simulink model "plant_harness"  (R2021a)
settings: Solver=ode4  StartTime=0.0  StopTime=10.0  FixedStep=0.001  RelTol=1e-3
undefined symbols (not defined in the file): DiscIntNeverNeededParam
libraries: vrlib x8, dspinverses x2, simulink x1, aerolibutil x1
settings Model: NumberOfSteps=10  Creator=jadg1  LastModifiedBy=jadg1

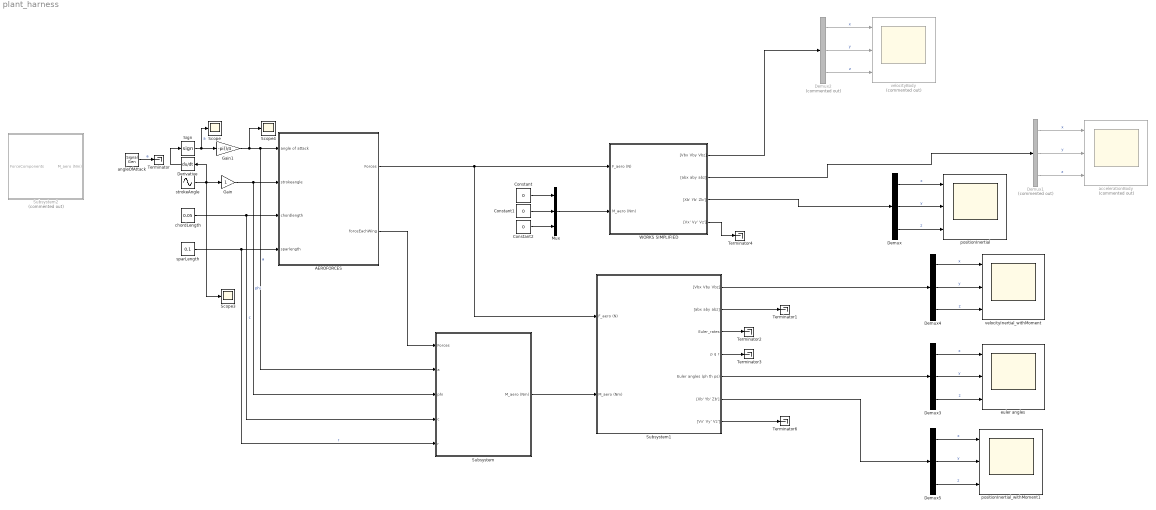
== system plant_harness ==
  AEROFORCES : Subsystem
  Constant : Constant  Value=0
  Constant1 : Constant  Value=0
  Constant2 : Constant  Value=0
  Demux{,3..5} (4 alike) : Demux  Outputs=3
  Demux1 : Demux  Commented=on  Outputs=3
  Demux2 : Demux  Commented=on  Outputs=3
  Derivative : Derivative
  Gain : Gain
  Gain1 : Gain  Gain=-pi()/4
  Mux : Mux  Inputs=3
  Scope : Scope
  Scope3 : Scope
  Scope4 : Scope
  Sign : Signum
  Subsystem : Subsystem
  Subsystem1 : Subsystem
  Subsystem2 : Subsystem  Commented=on
  Terminator{,1..4,6} (6 alike) : Terminator
  WORKS SIMPLIFIED : Subsystem
  accelerationBody : Scope  Commented=on  NumInputPorts=3
  angleOfAttack : SignalGenerator  WaveForm=square  Amplitude=pi()/6  Frequency=30
  chordLength : Constant  Value=0.05
  euler angles : Scope  NumInputPorts=3
  positionInertial : Scope  NumInputPorts=3
  positionInertial_withMoment1 : Scope  NumInputPorts=3
  sparLength : Constant  Value=0.1
  strokeAngle : Sin  Amplitude=pi()/2  Frequency=20*2*pi  Phase=pi()/2  SampleTime=0
  velocityBody : Scope  Commented=on  NumInputPorts=3
  velocityInertial_withMoment : Scope  NumInputPorts=3
  wires:
  sparLength/1 -> Subsystem/5(r), AEROFORCES/4(sparlength)  "r"
  chordLength/1 -> Subsystem/4(c), AEROFORCES/3(chordlength)  "c"
  Mux/1 -> WORKS SIMPLIFIED/2(M_aero (Nm))
  WORKS SIMPLIFIED/3("[Xb' Yb' Zb']") -> Demux/1
  WORKS SIMPLIFIED/4("[Vx' Vy' Vz']") -> Terminator4/1
  strokeAngle/1 -> Derivative/1, Scope3/1, Gain/1
  WORKS SIMPLIFIED/2("[abx aby abz]") -> Demux1/1
  WORKS SIMPLIFIED/1("[Vbx Vby Vbz]") -> Demux2/1
  Sign/1 -> Scope/1, Gain1/1  "a"
  Constant1/1 -> Mux/2
  Constant/1 -> Mux/1
  Constant2/1 -> Mux/3
  Demux/1 -> positionInertial/1  "x"
  Demux/2 -> positionInertial/2  "y"
  Demux/3 -> positionInertial/3  "z"
  Demux1/3 -> accelerationBody/3  "z"
  Demux1/2 -> accelerationBody/2  "y"
  Demux1/1 -> accelerationBody/1  "x"
  Demux2/1 -> velocityBody/1  "x"
  Demux2/2 -> velocityBody/2  "y"
  Demux2/3 -> velocityBody/3  "z"
  Demux3/3 -> euler angles/3  "z"
  Demux3/2 -> euler angles/2  "y"
  Demux3/1 -> euler angles/1  "x"
  Subsystem1/5(Euler angles (ph th ps)) -> Demux3/1
  Subsystem1/1("[Vbx Vby Vbz]") -> Demux4/1
  Subsystem1/2("[abx aby abz]") -> Terminator1/1
  Subsystem1/7("[Vx' Vy' Vz']") -> Terminator6/1
  Demux4/1 -> velocityInertial_withMoment/1  "x"
  Demux4/2 -> velocityInertial_withMoment/2  "y"
  Demux4/3 -> velocityInertial_withMoment/3  "z"
  Gain/1 -> Subsystem/3(phi), AEROFORCES/2(strokeangle)  "phi"
  Demux5/1 -> positionInertial_withMoment1/1  "x"
  Demux5/2 -> positionInertial_withMoment1/2  "y"
  Demux5/3 -> positionInertial_withMoment1/3  "z"
  Subsystem1/6("[Xb' Yb' Zb']") -> Demux5/1
  Subsystem1/3(Euler_rates) -> Terminator2/1
  Subsystem1/4(p q r) -> Terminator3/1
  Subsystem/1(M_aero (Nm)) -> Subsystem1/2(M_aero (Nm))
  AEROFORCES/2(forceEachWing) -> Subsystem/1(Forces)
  Gain1/1 -> Scope4/1, Subsystem/2(a), AEROFORCES/1(angle of attack)  "a"
  angleOfAttack/1 -> Terminator/1  "a"
  Derivative/1 -> Sign/1
  AEROFORCES/1(Forces) -> Subsystem1/1(F_aero (N)), WORKS SIMPLIFIED/1(F_aero (N))

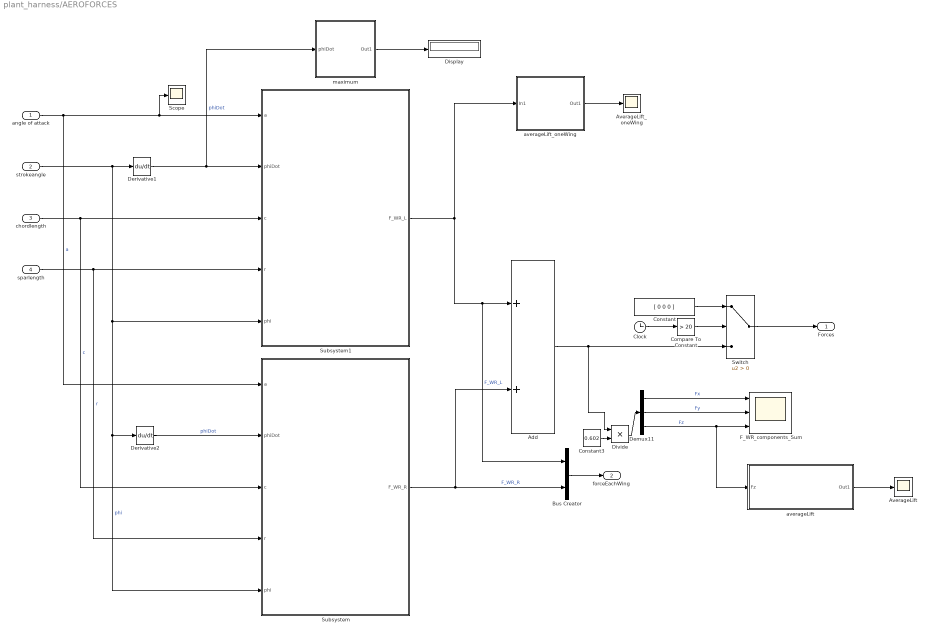
== system plant_harness/AEROFORCES ==
  angle of attack : Inport
  strokeangle : Inport  Port=2
  chordlength : Inport  Port=3
  sparlength : Inport  Port=4
  Add : Sum
  AverageLift : Scope
  AverageLift_oneWing : Scope
  Bus Creator : BusCreator  Inputs=2
  Clock : Clock
  Compare To Constant : simulink/Logic and Bit Operations/Compare To Constant  relop=>  const=20  OutDataTypeStr=boolean
  Constant : Constant  Value=[ 0 0 0 ]
  Constant3 : Constant  Value=0.602
  Demux11 : Demux  Outputs=3
  Derivative1 : Derivative
  Derivative2 : Derivative
  Display : Display
  Divide : Product  Inputs=**
  F_WR_components_Sum : Scope  NumInputPorts=3
  Scope : Scope
  Subsystem : Subsystem
  Subsystem1 : Subsystem
  Switch : Switch  Criteria=u2 > Threshold
  averageLift : Subsystem
  averageLift_oneWing : Subsystem
  maximum : Subsystem
  Forces : Outport
  forceEachWing : Outport  Port=2
  wires:
  Derivative1/1 -> maximum/1(phiDot), Subsystem1/2(phiDot)  "phiDot"
  Add/1 -> Divide/1, Switch/3
  Demux11/1 -> F_WR_components_Sum/1  "Fx"
  Demux11/3 -> F_WR_components_Sum/3, averageLift/1(Fz)  "Fz"
  Demux11/2 -> F_WR_components_Sum/2  "Fy"
  strokeangle/1 -> Subsystem/5(phi), Derivative2/1, Subsystem1/5(phi), Derivative1/1  "phi"
  chordlength/1 -> Subsystem/3(c), Subsystem1/3(c)  "c"
  sparlength/1 -> Subsystem/4(r), Subsystem1/4(r)  "r"
  Derivative2/1 -> Subsystem/2(phiDot)  "phiDot"
  Subsystem/1(F_WR_R) -> Add/2, Bus Creator/2  "F_WR_R"
  angle of attack/1 -> Subsystem/1(a), Scope/1, Subsystem1/1(a)  "a"
  Subsystem1/1(F_WR_L) -> averageLift_oneWing/1(In1), Bus Creator/1, Add/1  "F_WR_L"
  averageLift_oneWing/1(Out1) -> AverageLift_oneWing/1
  averageLift/1(Out1) -> AverageLift/1
  maximum/1(Out1) -> Display/1
  Switch/1 -> Forces/1
  Clock/1 -> Compare To Constant/1
  Compare To Constant/1 -> Switch/2
  Constant/1 -> Switch/1
  Bus Creator/1 -> forceEachWing/1
  Constant3/1 -> Divide/2
  Divide/1 -> Demux11/1

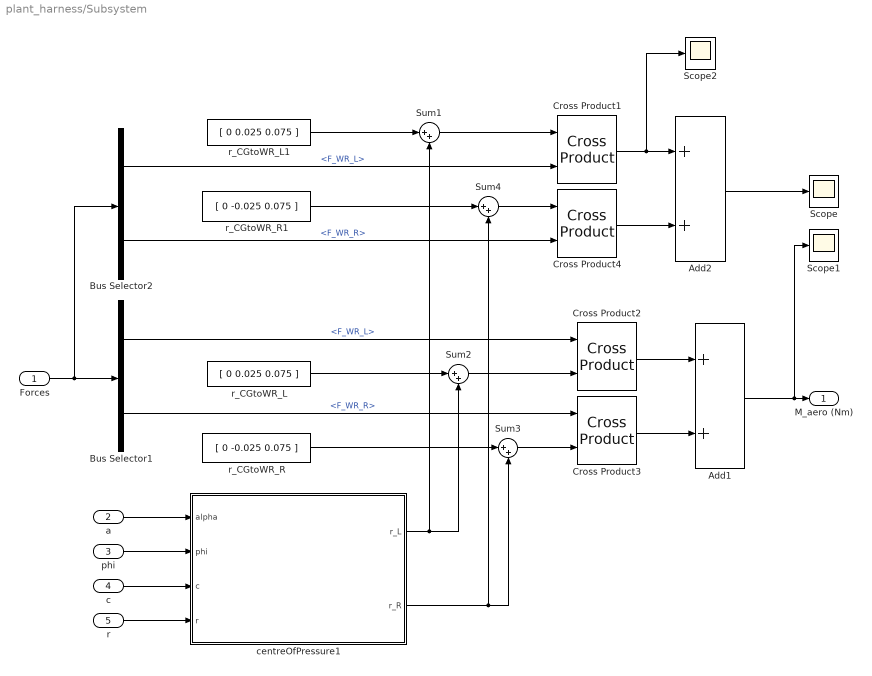
== system plant_harness/Subsystem ==
  Forces : Inport
  a : Inport  Port=2
  phi : Inport  Port=3
  c : Inport  Port=4
  r : Inport  Port=5
  Add1 : Sum
  Add2 : Sum
  Bus Selector1 : BusSelector  OutputSignals=F_WR_L,F_WR_R
  Bus Selector2 : BusSelector  OutputSignals=F_WR_L,F_WR_R
  Cross Product{1..4} (4 alike) : vrlib/Utilities/Cross Product
  Scope : Scope
  Scope1 : Scope
  Scope2 : Scope
  Sum{1..4} (4 alike) : Sum  Inputs=|++
  centreOfPressure1 : MATLAB Function  TreatAsAtomicUnit=on
  r_CGtoWR_L : Constant  Value=[ 0 0.025 0.075 ]
  r_CGtoWR_L1 : Constant  Value=[ 0 0.025 0.075 ]
  r_CGtoWR_R : Constant  Value=[ 0 -0.025 0.075 ]
  r_CGtoWR_R1 : Constant  Value=[ 0 -0.025 0.075 ]
  M_aero (Nm) : Outport
  wires:
  Bus Selector1/1 -> Cross Product2/1  "<F_WR_L>"
  r_CGtoWR_R/1 -> Sum3/1
  phi/1 -> centreOfPressure1/2(phi)
  centreOfPressure1/2(r_R) -> Sum4/2, Sum3/2
  Sum2/1 -> Cross Product2/2
  centreOfPressure1/1(r_L) -> Sum1/2, Sum2/2
  r/1 -> centreOfPressure1/4(r)
  c/1 -> centreOfPressure1/3(c)
  Sum3/1 -> Cross Product3/2
  Bus Selector1/2 -> Cross Product3/1  "<F_WR_R>"
  Add1/1 -> Scope1/1, M_aero (Nm)/1
  a/1 -> centreOfPressure1/1(alpha)
  Cross Product3/1 -> Add1/2
  Cross Product2/1 -> Add1/1
  Forces/1 -> Bus Selector2/1, Bus Selector1/1
  r_CGtoWR_L/1 -> Sum2/1
  Cross Product1/1 -> Scope2/1, Add2/1
  Cross Product4/1 -> Add2/2
  Bus Selector2/2 -> Cross Product4/2  "<F_WR_R>"
  Bus Selector2/1 -> Cross Product1/2  "<F_WR_L>"
  Sum1/1 -> Cross Product1/1
  r_CGtoWR_L1/1 -> Sum1/1
  Sum4/1 -> Cross Product4/1
  r_CGtoWR_R1/1 -> Sum4/1
  Add2/1 -> Scope/1

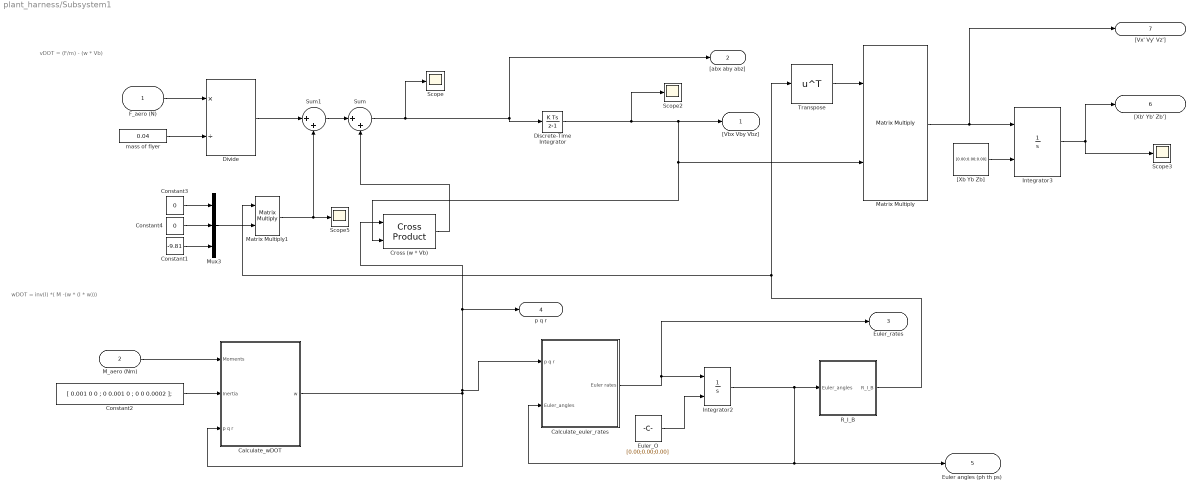
== system plant_harness/Subsystem1 ==
  note: wDOT = inv(I) *( M -(w * (I * w)))
  note: vDOT = (F/m) - (w * Vb)
  F_aero (N) : Inport
  M_aero (Nm) : Inport  Port=2
  Calculate_euler_rates : Subsystem
  Calculate_wDOT : Subsystem
  Constant1 : Constant  Value=-9.81
  Constant2 : Constant  Value=[ 0.001 0 0 ; 0 0.001 0 ; 0 0 0.0002 ];
  Constant3 : Constant  Value=0
  Constant4 : Constant  Value=0
  Cross (w * Vb) : vrlib/Utilities/Cross Product
  Discrete-Time Integrator : DiscreteIntegrator  SampleTime=-1  ICPrevOutput=DiscIntNeverNeededParam  ICPrevScaledInput=DiscIntNeverNeededParam
  Divide : Product  Inputs=*/
  Euler_O : Constant  Value=[0.00;0.00;0.00]
  Integrator2 : Integrator  InitialConditionSource=external
  Integrator3 : Integrator  InitialConditionSource=external
  Matrix Multiply : Product  Multiplication=Matrix(*)
  Matrix Multiply1 : Product  Multiplication=Matrix(*)
  Mux3 : Mux  Inputs=3
  R_I_B : Subsystem
  Scope{,2..3,5} (4 alike) : Scope
  Sum : Sum  Inputs=|++
  Sum1 : Sum  Inputs=|++
  Transpose : Math  Operator=transpose  SaturateOnIntegerOverflow=on
  "[Xb Yb Zb]" : Constant  Value=[0.00;0.00;0.00]
  mass of flyer : Constant  Value=0.04
  "[Vbx Vby Vbz]" : Outport
  "[abx aby abz]" : Outport  Port=2
  Euler_rates : Outport  Port=3
  p q r : Outport  Port=4
  Euler angles (ph th ps) : Outport  Port=5
  "[Xb' Yb' Zb']" : Outport  Port=6
  "[Vx' Vy' Vz']" : Outport  Port=7
  wires:
  Euler_O/1 -> Integrator2/2
  M_aero (Nm)/1 -> Calculate_wDOT/1(Moments)
  Calculate_euler_rates/1(Euler rates) -> Euler_rates/1, Integrator2/1
  F_aero (N)/1 -> Divide/1
  Transpose/1 -> Matrix Multiply/1
  "[Xb Yb Zb]"/1 -> Integrator3/2
  mass of flyer/1 -> Divide/2
  Calculate_wDOT/1(w) -> Calculate_wDOT/3(p q r), Cross (w * Vb)/1, p q r/1, Calculate_euler_rates/1(p q r)
  Constant2/1 -> Calculate_wDOT/2(Inertia)
  Matrix Multiply/1 -> "[Vx' Vy' Vz']"/1, Integrator3/1
  Discrete-Time Integrator/1 -> Scope2/1, "[Vbx Vby Vbz]"/1, Cross (w * Vb)/2, Matrix Multiply/2
  Integrator3/1 -> Scope3/1, "[Xb' Yb' Zb']"/1
  Cross (w * Vb)/1 -> Sum/2
  Integrator2/1 -> Calculate_euler_rates/2(Euler_angles), Euler angles (ph th ps)/1, R_I_B/1(Euler_angles)
  Sum/1 -> Scope/1, "[abx aby abz]"/1, Discrete-Time Integrator/1
  Constant4/1 -> Mux3/2
  Mux3/1 -> Matrix Multiply1/2
  Constant3/1 -> Mux3/1
  Matrix Multiply1/1 -> Sum1/2, Scope5/1
  Constant1/1 -> Mux3/3
  R_I_B/1(R_I_B) -> Matrix Multiply1/1, Transpose/1
  Divide/1 -> Sum1/1
  Sum1/1 -> Sum/1

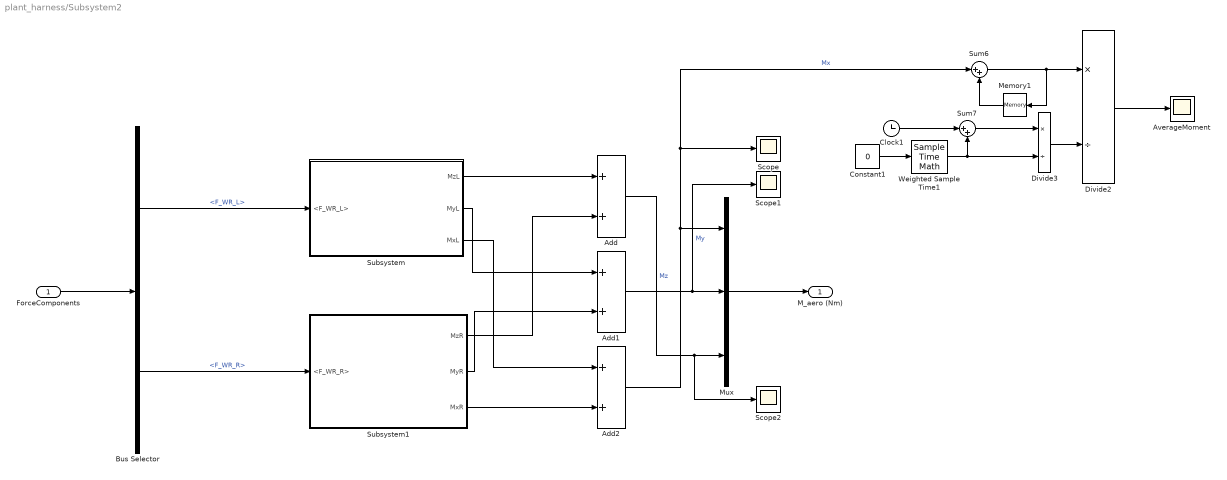
== system plant_harness/Subsystem2 ==
  ForceComponents : Inport
  Add : Sum
  Add1 : Sum
  Add2 : Sum
  AverageMoment : Scope
  Bus Selector : BusSelector  OutputSignals=F_WR_L,F_WR_R
  Clock1 : Clock
  Constant1 : Constant  Value=0
  Divide2 : Product  Inputs=*/
  Divide3 : Product  Inputs=*/
  Memory1 : Memory
  Mux : Mux  Inputs=3
  Scope : Scope
  Scope1 : Scope
  Scope2 : Scope
  Subsystem : Subsystem
  Subsystem1 : Subsystem
  Sum6 : Sum  Inputs=|++
  Sum7 : Sum  Inputs=|++
  Weighted Sample Time1 : SampleTimeMath  TsampMathOp=Ts Only
  M_aero (Nm) : Outport
  wires:
  ForceComponents/1 -> Bus Selector/1
  Bus Selector/1 -> Subsystem/1(<F_WR_L>)  "<F_WR_L>"
  Bus Selector/2 -> Subsystem1/1(<F_WR_R>)  "<F_WR_R>"
  Subsystem1/1(MzR) -> Add/2
  Subsystem/1(MzL) -> Add/1
  Subsystem1/2(MyR) -> Add1/2
  Subsystem/2(MyL) -> Add1/1
  Subsystem1/3(MxR) -> Add2/2
  Subsystem/3(MxL) -> Add2/1
  Add2/1 -> Sum6/1, Scope/1, Mux/1  "Mx"
  Add/1 -> Scope2/1, Mux/3  "Mz"
  Add1/1 -> Scope1/1, Mux/2  "My"
  Mux/1 -> M_aero (Nm)/1
  Weighted Sample Time1/1 -> Sum7/2, Divide3/2
  Sum6/1 -> Memory1/1, Divide2/1
  Constant1/1 -> Weighted Sample Time1/1
  Clock1/1 -> Sum7/1
  Divide3/1 -> Divide2/2
  Sum7/1 -> Divide3/1
  Divide2/1 -> AverageMoment/1
  Memory1/1 -> Sum6/2

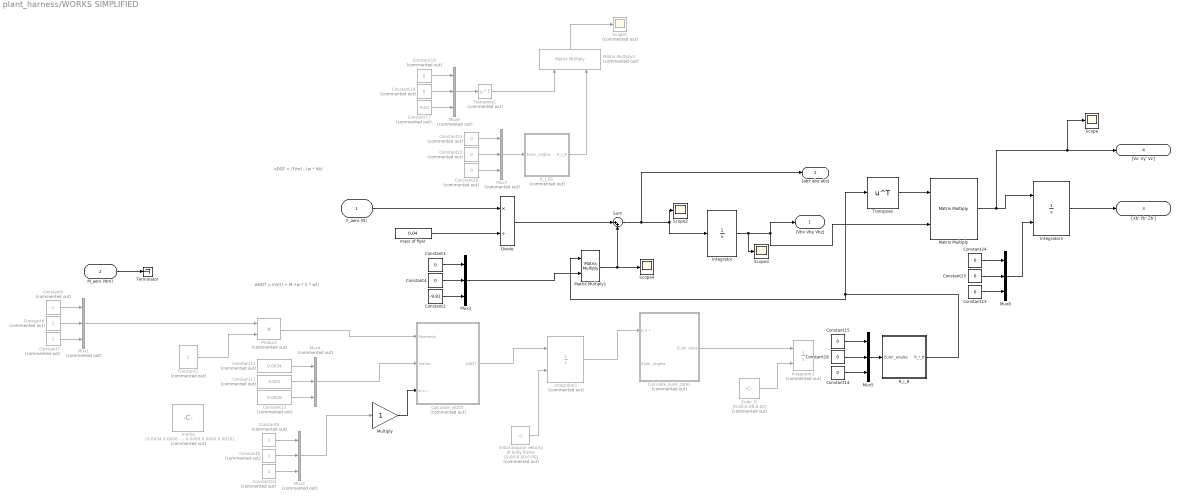
== system plant_harness/WORKS SIMPLIFIED ==
  note: wDOT = inv(I) + M -(w * (I * w))
  note: vDOT = (F/m) - (w * Vb)
  F_aero (N) : Inport
  M_aero (Nm) : Inport  Port=2
  Calculate_euler_rates : Subsystem  Commented=on
  Calculate_wDOT : Subsystem  Commented=on
  Constant{1,5..10} (7 alike) : Constant  Commented=on
  Constant11 : Constant  Commented=on  Value=0.001
  Constant12 : Constant  Commented=on  Value=0.0034
  Constant13 : Constant  Commented=on  Value=0.0026
  Constant{3..4,14..16,23..25} (8 alike) : Constant  Value=0
  Constant17 : Constant  Commented=on  Value=-9.81
  Constant{18..22} (5 alike) : Constant  Commented=on  Value=0
  Constant2 : Constant  Value=-9.81
  Divide : Product  Inputs=*/
  Euler_O : Constant  Commented=on  Value=[0.00;0.00;0.00]
  Inertia : Constant  Commented=on  Value=[0.0034 0.0000 0.0000; 0.0000 0.0010 0.0000; 0.0000 0.0000 0.0026]
  Initial angular velocity of body frame : Constant  Commented=on  Value=[0.00;0.00;0.00]
  Integrator : Integrator
  Integrator1 : Integrator  Commented=on  InitialConditionSource=external
  Integrator2 : Integrator  Commented=on  InitialConditionSource=external
  Integrator3 : Integrator  InitialConditionSource=external
  Matrix Multiply : Product  Multiplication=Matrix(*)
  Matrix Multiply1 : Product  Multiplication=Matrix(*)
  Matrix Multiply2 : Product  Commented=on  Multiplication=Matrix(*)
  Multiply : Gain
  Mux{1..2,4,6..7} (5 alike) : Mux  Commented=on  Inputs=3
  Mux3 : Mux  Inputs=3
  Mux5 : Mux  Inputs=3
  Mux8 : Mux  Inputs=3
  Product : Product  Commented=on
  R_I_B : Subsystem
  R_I_B1 : Subsystem  Commented=on
  Scope{,2..4} (4 alike) : Scope
  Scope1 : Scope  Commented=on
  Sum : Sum  Inputs=|++
  Terminator : Terminator
  Transpose : Math  Operator=transpose  SaturateOnIntegerOverflow=on
  Transpose1 : Math  Commented=on  Operator=transpose  SaturateOnIntegerOverflow=on
  mass of flyer : Constant  Value=0.04
  "[Vbx Vby Vbz]" : Outport
  "[abx aby abz]" : Outport  Port=2
  "[Xb' Yb' Zb']" : Outport  Port=3
  "[Vx' Vy' Vz']" : Outport  Port=4
  wires:
  mass of flyer/1 -> Divide/2
  M_aero (Nm)/1 -> Terminator/1
  Constant8/1 -> Mux2/1
  Euler_O/1 -> Integrator2/2
  Constant9/1 -> Mux2/2
  Product/1 -> Calculate_wDOT/1(Moments)
  F_aero (N)/1 -> Divide/1
  Constant13/1 -> Mux4/3
  Transpose/1 -> Matrix Multiply/1
  Initial angular velocity of body frame/1 -> Integrator1/2
  Integrator/1 -> Scope3/1, Matrix Multiply/2, "[Vbx Vby Vbz]"/1
  Integrator1/1 -> Calculate_euler_rates/1(p q r)
  Constant10/1 -> Mux2/3
  Mux4/1 -> Calculate_wDOT/2(Inertia)
  Constant12/1 -> Mux4/1
  Calculate_euler_rates/1(Euler rates) -> Integrator2/1
  Constant11/1 -> Mux4/2
  Mux2/1 -> Multiply/1
  Multiply/1 -> Calculate_wDOT/3(p q r)
  Matrix Multiply/1 -> "[Vx' Vy' Vz']"/1, Scope/1, Integrator3/1
  R_I_B/1(R_I_B) -> Transpose/1, Matrix Multiply1/1
  Constant1/1 -> Product/2
  Calculate_wDOT/1(wDOT) -> Integrator1/1
  Constant5/1 -> Mux1/1
  Constant6/1 -> Mux1/2
  Mux1/1 -> Product/1
  Constant7/1 -> Mux1/3
  Integrator3/1 -> "[Xb' Yb' Zb']"/1
  Constant16/1 -> Mux5/2
  Constant15/1 -> Mux5/1
  Mux5/1 -> R_I_B/1(Euler_angles)
  Constant14/1 -> Mux5/3
  Divide/1 -> Sum/1
  Sum/1 -> "[abx aby abz]"/1, Scope2/1, Integrator/1
  Constant2/1 -> Mux3/3
  Constant3/1 -> Mux3/1
  Constant4/1 -> Mux3/2
  Constant18/1 -> Mux6/1
  Constant19/1 -> Mux6/2
  Constant17/1 -> Mux6/3
  Constant20/1 -> Mux7/3
  Constant21/1 -> Mux7/1
  Constant22/1 -> Mux7/2
  Matrix Multiply2/1 -> Scope1/1
  Mux7/1 -> R_I_B1/1(Euler_angles)
  Mux6/1 -> Transpose1/1
  Transpose1/1 -> Matrix Multiply2/1
  R_I_B1/1(R_I_B) -> Matrix Multiply2/2
  Matrix Multiply1/1 -> Scope4/1, Sum/2
  Mux3/1 -> Matrix Multiply1/2
  Mux8/1 -> Integrator3/2
  Constant23/1 -> Mux8/3
  Constant25/1 -> Mux8/2
  Constant24/1 -> Mux8/1

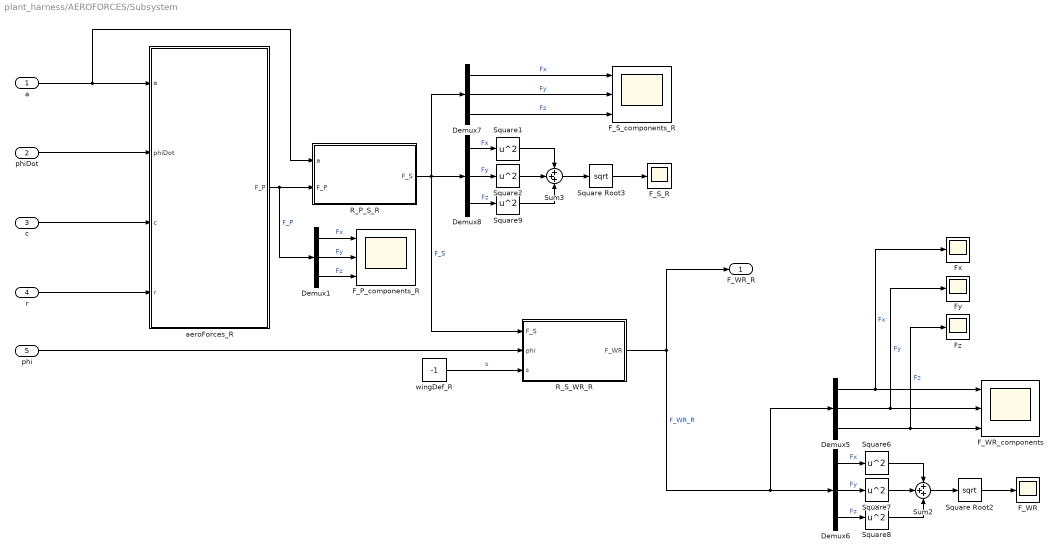
== system plant_harness/AEROFORCES/Subsystem ==
  a : Inport
  phiDot : Inport  Port=2
  c : Inport  Port=3
  r : Inport  Port=4
  phi : Inport  Port=5
  Demux{1,5..8} (5 alike) : Demux  Outputs=3
  F_P_components_R : Scope  NumInputPorts=3
  F_S_R : Scope
  F_S_components_R : Scope  NumInputPorts=3
  F_WR : Scope
  F_WR_components : Scope  NumInputPorts=3
  Fx : Scope
  Fy : Scope
  Fz : Scope
  R_P_S_R : MATLAB Function  TreatAsAtomicUnit=on
  R_S_WR_R : MATLAB Function  TreatAsAtomicUnit=on
  Square Root2 : Sqrt  SaturateOnIntegerOverflow=on
  Square Root3 : Sqrt  SaturateOnIntegerOverflow=on
  Square{1..2,6..9} (6 alike) : Math  Operator=square  SaturateOnIntegerOverflow=on
  Sum2 : Sum  Inputs=+++
  Sum3 : Sum  Inputs=+++
  aeroForces_R : MATLAB Function  TreatAsAtomicUnit=on
  wingDef_R : Constant  Value=-1
  F_WR_R : Outport
  wires:
  Demux8/3 -> Square9/1  "Fz"
  Square9/1 -> Sum3/3
  aeroForces_R/1(F_P) -> R_P_S_R/2(F_P), Demux1/1  "F_P"
  a/1 -> aeroForces_R/1(a), R_P_S_R/1(a)
  R_P_S_R/1(F_S) -> Demux8/1, Demux7/1, R_S_WR_R/1(F_S)  "F_S"
  r/1 -> aeroForces_R/4(r)
  Demux8/1 -> Square1/1  "Fx"
  phi/1 -> R_S_WR_R/2(phi)
  Square1/1 -> Sum3/1
  Demux8/2 -> Square2/1  "Fy"
  Demux7/3 -> F_S_components_R/3  "Fz"
  Demux7/2 -> F_S_components_R/2  "Fy"
  Demux1/2 -> F_P_components_R/2  "Fy"
  Demux1/1 -> F_P_components_R/1  "Fx"
  c/1 -> aeroForces_R/3(c)
  Demux7/1 -> F_S_components_R/1  "Fx"
  Sum3/1 -> Square Root3/1
  phiDot/1 -> aeroForces_R/2(phiDot)
  Square2/1 -> Sum3/2
  Demux1/3 -> F_P_components_R/3  "Fz"
  Square Root3/1 -> F_S_R/1
  wingDef_R/1 -> R_S_WR_R/3(s)  "s"
  R_S_WR_R/1(F_WR) -> Demux5/1, Demux6/1, F_WR_R/1  "F_WR_R"
  Square Root2/1 -> F_WR/1
  Demux5/3 -> Fz/1, F_WR_components/3  "Fz"
  Demux5/2 -> F_WR_components/2, Fy/1  "Fy"
  Square7/1 -> Sum2/2
  Square8/1 -> Sum2/3
  Demux5/1 -> Fx/1, F_WR_components/1  "Fx"
  Sum2/1 -> Square Root2/1
  Demux6/2 -> Square7/1  "Fy"
  Square6/1 -> Sum2/1
  Demux6/1 -> Square6/1  "Fx"
  Demux6/3 -> Square8/1  "Fz"

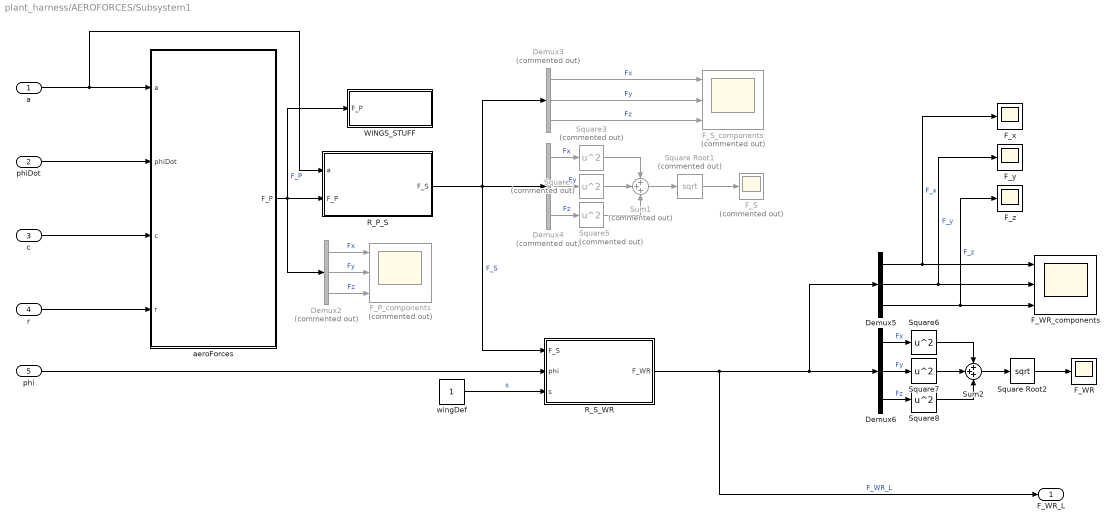
== system plant_harness/AEROFORCES/Subsystem1 ==
  a : Inport
  phiDot : Inport  Port=2
  c : Inport  Port=3
  r : Inport  Port=4
  phi : Inport  Port=5
  Demux2 : Demux  Commented=on  Outputs=3
  Demux3 : Demux  Commented=on  Outputs=3
  Demux4 : Demux  Commented=on  Outputs=3
  Demux5 : Demux  Outputs=3
  Demux6 : Demux  Outputs=3
  F_P_components : Scope  Commented=on  NumInputPorts=3
  F_S : Scope  Commented=on
  F_S_components : Scope  Commented=on  NumInputPorts=3
  F_WR : Scope
  F_WR_components : Scope  NumInputPorts=3
  F_x : Scope
  F_y : Scope
  F_z : Scope
  R_P_S : MATLAB Function  TreatAsAtomicUnit=on
  R_S_WR : MATLAB Function  TreatAsAtomicUnit=on
  Square Root1 : Sqrt  Commented=on  SaturateOnIntegerOverflow=on
  Square Root2 : Sqrt  SaturateOnIntegerOverflow=on
  Square3 : Math  Commented=on  Operator=square  SaturateOnIntegerOverflow=on
  Square4 : Math  Commented=on  Operator=square  SaturateOnIntegerOverflow=on
  Square5 : Math  Commented=on  Operator=square  SaturateOnIntegerOverflow=on
  Square6 : Math  Operator=square  SaturateOnIntegerOverflow=on
  Square7 : Math  Operator=square  SaturateOnIntegerOverflow=on
  Square8 : Math  Operator=square  SaturateOnIntegerOverflow=on
  Sum1 : Sum  Commented=on  Inputs=+++
  Sum2 : Sum  Inputs=+++
  WINGS_STUFF : Subsystem
  aeroForces : MATLAB Function  TreatAsAtomicUnit=on
  wingDef : Constant
  F_WR_L : Outport
  wires:
  Demux2/3 -> F_P_components/3  "Fz"
  wingDef/1 -> R_S_WR/3(s)  "s"
  Square6/1 -> Sum2/1
  phiDot/1 -> aeroForces/2(phiDot)
  Square7/1 -> Sum2/2
  Demux6/3 -> Square8/1  "Fz"
  Demux4/3 -> Square5/1  "Fz"
  aeroForces/1(F_P) -> WINGS_STUFF/1(F_P), Demux2/1, R_P_S/2(F_P)  "F_P"
  Demux2/1 -> F_P_components/1  "Fx"
  Demux5/3 -> F_z/1, F_WR_components/3  "F_z"
  Demux6/1 -> Square6/1  "Fx"
  Demux3/3 -> F_S_components/3  "Fz"
  R_S_WR/1(F_WR) -> F_WR_L/1, Demux5/1, Demux6/1  "F_WR_L"
  R_P_S/1(F_S) -> R_S_WR/1(F_S), Demux3/1, Demux4/1  "F_S"
  Demux3/2 -> F_S_components/2  "Fy"
  Square4/1 -> Sum1/2
  Demux6/2 -> Square7/1  "Fy"
  r/1 -> aeroForces/4(r)
  Sum2/1 -> Square Root2/1
  Demux5/1 -> F_x/1, F_WR_components/1  "F_x"
  Demux4/2 -> Square4/1  "Fy"
  Square8/1 -> Sum2/3
  Square5/1 -> Sum1/3
  Demux5/2 -> F_WR_components/2, F_y/1  "F_y"
  Square3/1 -> Sum1/1
  a/1 -> R_P_S/1(a), aeroForces/1(a)
  Square Root1/1 -> F_S/1
  Demux3/1 -> F_S_components/1  "Fx"
  Demux2/2 -> F_P_components/2  "Fy"
  Sum1/1 -> Square Root1/1
  Demux4/1 -> Square3/1  "Fx"
  Square Root2/1 -> F_WR/1
  c/1 -> aeroForces/3(c)
  phi/1 -> R_S_WR/2(phi)

== system plant_harness/AEROFORCES/averageLift ==
  Fz : Inport
  Clock : Clock
  Constant : Constant  Value=0
  Divide : Product  Inputs=*/
  Divide1 : Product  Inputs=*/
  Memory : Memory
  Sum : Sum  Inputs=|++
  Sum5 : Sum  Inputs=|++
  Weighted Sample Time : SampleTimeMath  TsampMathOp=Ts Only
  Out1 : Outport
  wires:
  Sum/1 -> Memory/1, Divide/1
  Weighted Sample Time/1 -> Sum5/2, Divide1/2
  Memory/1 -> Sum/2
  Divide1/1 -> Divide/2
  Fz/1 -> Sum/1
  Divide/1 -> Out1/1
  Constant/1 -> Weighted Sample Time/1
  Clock/1 -> Sum5/1
  Sum5/1 -> Divide1/1

== system plant_harness/AEROFORCES/averageLift_oneWing ==
  In1 : Inport
  Clock1 : Clock
  Constant1 : Constant  Value=0
  Divide2 : Product  Inputs=*/
  Divide3 : Product  Inputs=*/
  Memory1 : Memory
  Sum6 : Sum  Inputs=|++
  Sum7 : Sum  Inputs=|++
  Weighted Sample Time1 : SampleTimeMath  TsampMathOp=Ts Only
  Out1 : Outport
  wires:
  Weighted Sample Time1/1 -> Sum7/2, Divide3/2
  Sum7/1 -> Divide3/1
  Clock1/1 -> Sum7/1
  Divide3/1 -> Divide2/2
  Constant1/1 -> Weighted Sample Time1/1
  Sum6/1 -> Memory1/1, Divide2/1
  Memory1/1 -> Sum6/2
  Divide2/1 -> Out1/1
  In1/1 -> Sum6/1

== system plant_harness/AEROFORCES/maximum ==
  phiDot : Inport
  GreaterThan : RelationalOperator  Operator=>  OutDataTypeStr=boolean  RndMeth=Simplest
  Memory2 : Memory
  Switch : Switch  Criteria=u2 > Threshold
  Out1 : Outport
  wires:
  Switch/1 -> Out1/1, Memory2/1
  phiDot/1 -> GreaterThan/1, Switch/1
  Memory2/1 -> Switch/3, GreaterThan/2
  GreaterThan/1 -> Switch/2

== system plant_harness/Subsystem1/Calculate_euler_rates ==
  note: psi dot
  note: theta dot
  note: phi dot
  note: psi
  p q r : Inport
  Euler_angles : Inport  Port=2
  Calc_my_euler_rates : MATLAB Function  TreatAsAtomicUnit=on
  Demux : Demux  Outputs=[-1;1;1]
  Demux1 : Demux  Outputs=[1;1;1]
  Demux2 : Demux  Outputs=3
  Mux : Mux  Inputs=3
  Terminator : Terminator
  Euler rates : Outport
  wires:
  Demux/1 -> Terminator/1
  Euler_angles/1 -> Demux/1
  Demux/2 -> Calc_my_euler_rates/1(theta)
  Demux/3 -> Calc_my_euler_rates/2(phi)
  p q r/1 -> Demux1/1
  Demux1/2 -> Calc_my_euler_rates/4(q)
  Demux1/1 -> Calc_my_euler_rates/3(p)
  Demux1/3 -> Calc_my_euler_rates/5(r)
  Calc_my_euler_rates/1(euler_rates) -> Demux2/1
  Demux2/2 -> Mux/2
  Demux2/1 -> Mux/1
  Demux2/3 -> Mux/3
  Mux/1 -> Euler rates/1

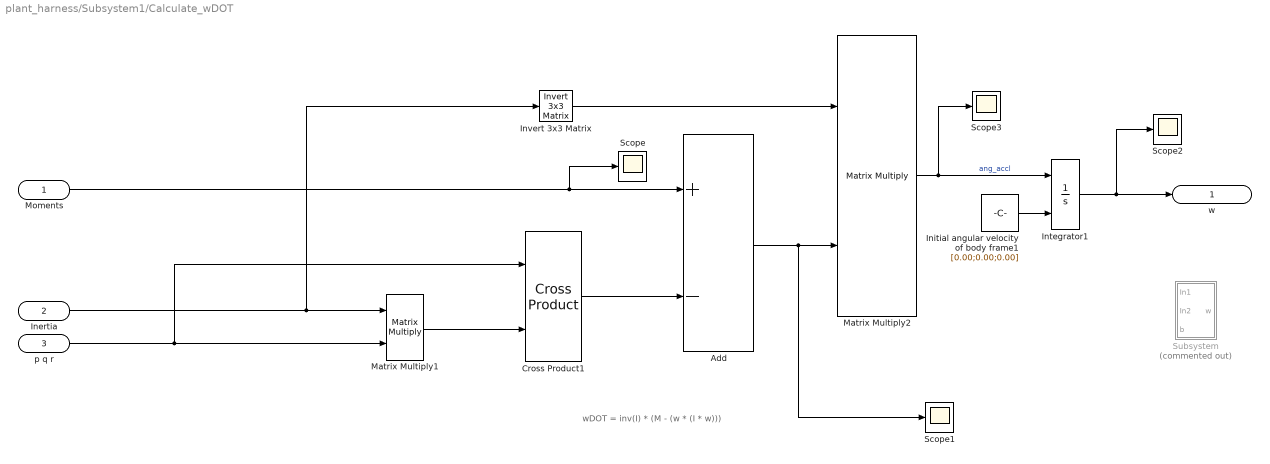
== system plant_harness/Subsystem1/Calculate_wDOT ==
  note: wDOT = inv(I) * (M - (w * (I * w)))
  Moments : Inport
  Inertia : Inport  Port=2
  p q r : Inport  Port=3
  Add : Sum  Inputs=+-
  Cross Product1 : vrlib/Utilities/Cross Product
  Initial angular velocity of body frame1 : Constant  Value=[0.00;0.00;0.00]
  Integrator1 : Integrator  InitialConditionSource=external
  Invert 3x3 Matrix : aerolibutil/Invert  3x3 Matrix
  Matrix Multiply1 : Product  Multiplication=Matrix(*)
  Matrix Multiply2 : Product  Multiplication=Matrix(*)
  Scope{,1..3} (4 alike) : Scope
  Subsystem : Subsystem  Commented=on
  w : Outport
  wires:
  Inertia/1 -> Invert 3x3 Matrix/1, Matrix Multiply1/1
  p q r/1 -> Cross Product1/1, Matrix Multiply1/2
  Matrix Multiply1/1 -> Cross Product1/2
  Cross Product1/1 -> Add/2
  Moments/1 -> Scope/1, Add/1
  Add/1 -> Scope1/1, Matrix Multiply2/2
  Invert 3x3 Matrix/1 -> Matrix Multiply2/1
  Matrix Multiply2/1 -> Scope3/1, Integrator1/1  "ang_accl"
  Initial angular velocity of body frame1/1 -> Integrator1/2
  Integrator1/1 -> Scope2/1, w/1

== system plant_harness/Subsystem1/R_I_B ==
  Euler_angles : Inport
  Demux : Demux  Outputs=[1;1;1]
  MATLAB Function : MATLAB Function  TreatAsAtomicUnit=on
  R_I_B : Outport
  wires:
  Euler_angles/1 -> Demux/1
  Demux/2 -> MATLAB Function/2(theta)
  Demux/3 -> MATLAB Function/3(psi)
  Demux/1 -> MATLAB Function/1(phi)
  MATLAB Function/1(R_I_B) -> R_I_B/1

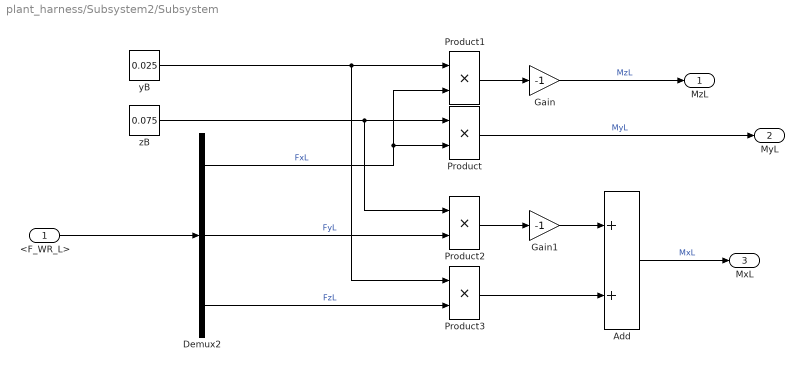
== system plant_harness/Subsystem2/Subsystem ==
  <F_WR_L> : Inport
  Add : Sum
  Demux2 : Demux  Outputs=3
  Gain : Gain  Gain=-1
  Gain1 : Gain  Gain=-1
  Product{,1..3} (4 alike) : Product
  yB : Constant  Value=0.025
  zB : Constant  Value=0.075
  MzL : Outport
  MyL : Outport  Port=2
  MxL : Outport  Port=3
  wires:
  yB/1 -> Product3/1, Product1/1
  Gain1/1 -> Add/1
  Product1/1 -> Gain/1
  Product3/1 -> Add/2
  Demux2/1 -> Product1/2, Product/2  "FxL"
  Demux2/3 -> Product3/2  "FzL"
  Product/1 -> MyL/1  "MyL"
  Demux2/2 -> Product2/2  "FyL"
  zB/1 -> Product2/1, Product/1
  Product2/1 -> Gain1/1
  <F_WR_L>/1 -> Demux2/1
  Add/1 -> MxL/1  "MxL"
  Gain/1 -> MzL/1  "MzL"

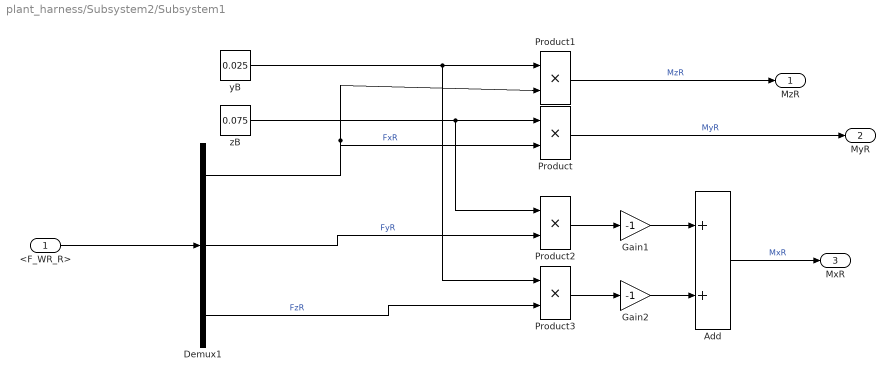
== system plant_harness/Subsystem2/Subsystem1 ==
  <F_WR_R> : Inport
  Add : Sum
  Demux1 : Demux  Outputs=3
  Gain1 : Gain  Gain=-1
  Gain2 : Gain  Gain=-1
  Product{,1..3} (4 alike) : Product
  yB : Constant  Value=0.025
  zB : Constant  Value=0.075
  MzR : Outport
  MyR : Outport  Port=2
  MxR : Outport  Port=3
  wires:
  Demux1/1 -> Product1/2, Product/2  "FxR"
  Demux1/2 -> Product2/2  "FyR"
  Demux1/3 -> Product3/2  "FzR"
  <F_WR_R>/1 -> Demux1/1
  zB/1 -> Product2/1, Product/1
  Product2/1 -> Gain1/1
  Product3/1 -> Gain2/1
  yB/1 -> Product3/1, Product1/1
  Gain1/1 -> Add/1
  Product/1 -> MyR/1  "MyR"
  Product1/1 -> MzR/1  "MzR"
  Add/1 -> MxR/1  "MxR"
  Gain2/1 -> Add/2

== system plant_harness/WORKS SIMPLIFIED/Calculate_euler_rates ==
  note: ps dot
  note: th dot
  note: ph dot
  note: ph
  p q r : Inport
  Euler_angles : Inport  Port=2
  Calc_my_euler_rates : MATLAB Function  TreatAsAtomicUnit=on
  Demux : Demux  Outputs=[-1;1;1]
  Demux1 : Demux  Outputs=[1;1;1]
  Demux2 : Demux  Outputs=3
  Mux : Mux  Inputs=3
  Terminator : Terminator
  Euler rates : Outport
  wires:
  Demux/1 -> Terminator/1
  Euler_angles/1 -> Demux/1
  Demux/2 -> Calc_my_euler_rates/1(th)
  Demux/3 -> Calc_my_euler_rates/2(ps)
  p q r/1 -> Demux1/1
  Demux1/2 -> Calc_my_euler_rates/4(q)
  Demux1/1 -> Calc_my_euler_rates/3(p)
  Demux1/3 -> Calc_my_euler_rates/5(r)
  Calc_my_euler_rates/1(euler_rates) -> Demux2/1
  Demux2/2 -> Mux/2
  Demux2/1 -> Mux/1
  Demux2/3 -> Mux/3
  Mux/1 -> Euler rates/1

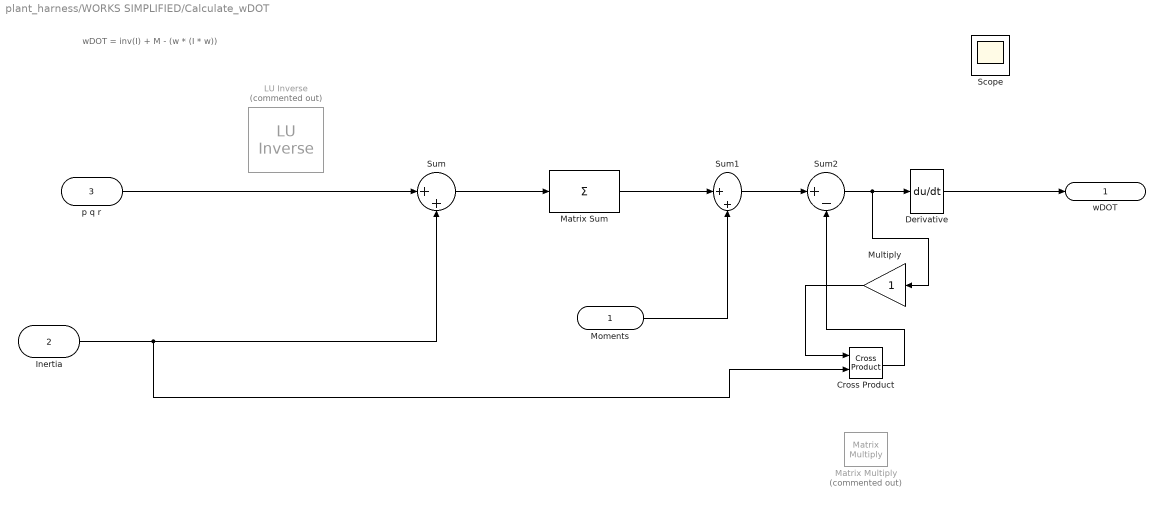
== system plant_harness/WORKS SIMPLIFIED/Calculate_wDOT ==
  note: wDOT = inv(I) + M - (w * (I * w))
  Moments : Inport
  Inertia : Inport  Port=2
  p q r : Inport  Port=3
  " LU Inverse" : dspinverses/ LU Inverse  Commented=on
  Cross Product : vrlib/Utilities/Cross Product
  Derivative : Derivative
  Matrix Sum : Sum  Inputs=+
  Matrix Multiply : Product  Commented=on  Multiplication=Matrix(*)
  Multiply : Gain
  Scope : Scope
  Sum : Sum  Inputs=|++
  Sum1 : Sum  Inputs=|++
  Sum2 : Sum  Inputs=|+-
  wDOT : Outport
  wires:
  Sum/1 -> Matrix Sum/1
  Matrix Sum/1 -> Sum1/1
  Sum1/1 -> Sum2/1
  Multiply/1 -> Cross Product/1
  Sum2/1 -> Multiply/1, Derivative/1
  Cross Product/1 -> Sum2/2
  Derivative/1 -> wDOT/1
  Moments/1 -> Sum1/2
  p q r/1 -> Sum/1
  Inertia/1 -> Cross Product/2, Sum/2

== system plant_harness/WORKS SIMPLIFIED/R_I_B ==
  Euler_angles : Inport
  Demux : Demux  Outputs=[1;1;1]
  MATLAB Function : MATLAB Function  TreatAsAtomicUnit=on
  R_I_B : Outport
  wires:
  Euler_angles/1 -> Demux/1
  Demux/2 -> MATLAB Function/2(th)
  Demux/3 -> MATLAB Function/3(ps)
  Demux/1 -> MATLAB Function/1(ph)
  MATLAB Function/1(R_I_B) -> R_I_B/1

== system plant_harness/WORKS SIMPLIFIED/R_I_B1 ==
  Euler_angles : Inport
  Demux : Demux  Outputs=[1;1;1]
  MATLAB Function : MATLAB Function  TreatAsAtomicUnit=on
  R_I_B : Outport
  wires:
  Euler_angles/1 -> Demux/1
  Demux/2 -> MATLAB Function/2(th)
  Demux/3 -> MATLAB Function/3(ps)
  Demux/1 -> MATLAB Function/1(ph)
  MATLAB Function/1(R_I_B) -> R_I_B/1

== system plant_harness/AEROFORCES/Subsystem1/WINGS_STUFF ==
  F_P : Inport
  Demux4 : Demux  Outputs=3
  Display : Display
  GreaterThan : RelationalOperator  Operator=>  OutDataTypeStr=boolean  RndMeth=Simplest
  Memory1 : Memory
  Square Root1 : Sqrt  SaturateOnIntegerOverflow=on
  Square3 : Math  Operator=square  SaturateOnIntegerOverflow=on
  Square4 : Math  Operator=square  SaturateOnIntegerOverflow=on
  Square5 : Math  Operator=square  SaturateOnIntegerOverflow=on
  Sum1 : Sum  Inputs=+++
  Switch : Switch  Criteria=u2 > Threshold
  Total Force Over Time : Scope
  wires:
  Square3/1 -> Sum1/1
  Sum1/1 -> Square Root1/1
  Square4/1 -> Sum1/2
  Demux4/2 -> Square4/1  "Fy"
  Demux4/3 -> Square5/1  "Fz"
  Square5/1 -> Sum1/3
  Demux4/1 -> Square3/1  "Fx"
  F_P/1 -> Demux4/1
  Square Root1/1 -> GreaterThan/1, Switch/1, Total Force Over Time/1  "Total Force"
  Memory1/1 -> Switch/3, GreaterThan/2
  GreaterThan/1 -> Switch/2
  Switch/1 -> Display/1, Memory1/1

== system plant_harness/Subsystem1/Calculate_wDOT/Subsystem ==
  In1 : Inport
  In2 : Inport  Port=2
  b : Inport  Port=3
  " LU Inverse" : dspinverses/ LU Inverse  Commented=on
  Cross Product : vrlib/Utilities/Cross Product
  Initial angular velocity of body frame : Constant  Value=[0.00;0.00;0.00]
  Integrator : Integrator  InitialConditionSource=external
  Matrix Multiply : Product  Commented=on  Multiplication=Matrix(*)
  Multiply : Gain
  Sum : Sum  Inputs=|++
  Sum1 : Sum  Inputs=|++
  Sum2 : Sum  Inputs=|+-
  w : Outport
  wires:
  Sum2/1 -> Integrator/1
  b/1 -> Cross Product/2, Sum/2
  Sum/1 -> Sum1/1
  Cross Product/1 -> Sum2/2
  Integrator/1 -> w/1, Multiply/1
  Initial angular velocity of body frame/1 -> Integrator/2
  Sum1/1 -> Sum2/1
  Multiply/1 -> Cross Product/1
  In1/1 -> Sum/1
  In2/1 -> Sum1/2

== matlab function plant_harness/Subsystem1/Calculate_euler_rates/Calc_my_euler_rates ==
  data: theta input; euler_rates output; phi input; p input; q input; r input
function euler_rates = my_euler_rates(theta,phi,p,q,r) 

 euler_rates = [        r - p*sin(theta)              ;
                 q*cos(phi) + p*cos(theta)*sin(phi)   ;
                 p*cos(phi)*cos(theta) - q*sin(phi)   ;
               ];
           
end

== matlab function plant_harness/Subsystem1/R_I_B/MATLAB Function ==
  data: phi input; R_I_B output; theta input; psi input
function R_I_B = calc_R_I_B(phi, theta, psi)

R_I_B = [                  cos(theta)*cos(psi)                               -cos(theta)*sin(psi)                         sin(theta)     ;
               sin(phi)*sin(theta)*cos(psi)+cos(phi)*sin(psi)    -sin(phi)*sin(theta)*sin(psi)+cos(phi)*cos(psi)    -sin(phi)*cos(theta) ;
              -cos(phi)*sin(theta)*cos(psi)+sin(phi)*sin(psi)     cos(phi)*sin(theta)*sin(psi)+sin(phi)*cos(psi)     cos(phi)*cos(theta) ;
        ];
end

== matlab function plant_harness/AEROFORCES/Subsystem1/R_S_WR ==
  data: F_S input; phi input; s input; F_WR output
function F_WR = S_to_WR(F_S,phi,s)

arg = s*phi;

R_S_WR = [  
           cos(arg)  -sin(arg)    0 ;
           sin(arg)   cos(arg)    0 ;
              0          0        1 ;
         ];

F_WR = R_S_WR * F_S;

end

== matlab function plant_harness/AEROFORCES/Subsystem1/aeroForces ==
  data: a input; F_P output; phiDot input; c input; r input
function F_P = aeroForces(a,phiDot,c,r)

% Declare sizes
F_P = zeros(3,1);

% Define the density of air [kg/m^3]
p = 1.225; 

% Define the value of the F-P angle theta
theta = -a;

% Define the lift and drag coefficients using the absolute value of alpha
cL = 0.225 + 1.58*sin((2.13*abs(a))-(7.2*(pi()/180)));
cD = 1.92 - 1.55*cos((2.04*abs(a))-(9.82*(pi()/180)));

% Calculate the cartesian components of the force vector in the P frame
Fx_P = (-1/6)*cos(theta)*sign(a)*p*(phiDot^2)*cD*c*(r^3) + (1/6)*sin(theta)*p*(phiDot^2)*cL*c*(r^3);
Fy_P = 0;
Fz_P = (1/6)*sin(theta)*sign(a)*p*(phiDot^2)*cD*c*(r^3) + (1/6)*cos(theta)*p*(phiDot^2)*cL*c*(r^3);

% Construct the force vector in the P frame
F_P = [ Fx_P ;
        Fy_P ; 
        Fz_P ; ];

end

== matlab function plant_harness/AEROFORCES/Subsystem1/R_P_S ==
  data: a input; F_P input; F_S output
function F_S = P_to_S(a,F_P)

R_P_S = [  
           cos(a)   0   sin(a) ;
             0      1     0    ;
          -sin(a)   0   cos(a) ;
        ];

F_S = R_P_S * F_P;

end

== matlab function plant_harness/AEROFORCES/Subsystem/R_P_S_R ==
  data: a input; F_P input; F_S output
function F_S = P_to_S(a,F_P)

R_P_S = [  
           cos(a)   0   sin(a) ;
             0      1     0    ;
          -sin(a)   0   cos(a) ;
        ];

F_S = R_P_S * F_P;

end

== matlab function plant_harness/AEROFORCES/Subsystem/R_S_WR_R ==
  data: F_S input; phi input; s input; F_WR output
function F_WR = S_to_WR(F_S,phi,s)

arg = s*phi;

R_S_WR = [  
           cos(arg)  -sin(arg)    0 ;
           sin(arg)   cos(arg)    0 ;
              0          0        1 ;
         ];

F_WR = R_S_WR * F_S;

end

== matlab function plant_harness/AEROFORCES/Subsystem/aeroForces_R ==
  data: a input; F_P output; phiDot input; c input; r input
function F_P = aeroForces(a,phiDot,c,r)

% Declare sizes
F_P = zeros(3,1);

% Define the density of air [kg/m^3]
p = 1.225; 

% Define the value of the F-P angle theta
theta = -a;

% Define the lift and drag coefficients using the absolute value of alpha
cL = 0.225 + 1.58*sin((2.13*abs(a))-(7.2*(pi()/180)));
cD = 1.92 - 1.55*cos((2.04*abs(a))-(9.82*(pi()/180)));

% Calculate the cartesian components of the force vector in the P frame
Fx_P = (-1/6)*cos(theta)*sign(a)*p*(phiDot^2)*cD*c*(r^3) + (1/6)*sin(theta)*p*(phiDot^2)*cL*c*(r^3);
Fy_P = 0;
Fz_P = (1/6)*sin(theta)*sign(a)*p*(phiDot^2)*cD*c*(r^3) + (1/6)*cos(theta)*p*(phiDot^2)*cL*c*(r^3);

% Construct the force vector in the P frame
F_P = [ Fx_P ;
        Fy_P ; 
        Fz_P ; ];

end

== matlab function plant_harness/WORKS SIMPLIFIED/Calculate_euler_rates/Calc_my_euler_rates ==
  data: th input; euler_rates output; ps input; p input; q input; r input
function euler_rates = my_euler_rates(th,ps,p,q,r)
euler_rates = [(r .* cos(ps) + q .* sin(ps)) ./ cos(th);
                q .* cos(ps) - r .* sin(ps);
                (p .* cos(th) + r.* cos(ps) .* sin(th) + q .* sin(ps) .* sin(th)) ./ cos(th)];
end

== matlab function plant_harness/WORKS SIMPLIFIED/R_I_B/MATLAB Function ==
  data: ph input; R_I_B output; th input; ps input
function R_I_B = calc_R_I_B(ph, th, ps)

R_I_B = [cos(th)*cos(ps)              cos(th)*sin(ps)              -sin(th);
               sin(ph)*sin(th)*cos(ps)-cos(ph)*sin(ps)  sin(ph)*sin(th)*sin(ps)+cos(ph)*cos(ps)  sin(ph)*cos(th);
               cos(ph)*sin(th)*cos(ps)+sin(ph)*sin(ps)  cos(ph)*sin(th)*sin(ps)-sin(ph)*cos(ps)  cos(ph)*cos(th)];
end

== matlab function plant_harness/WORKS SIMPLIFIED/R_I_B1/MATLAB Function ==
  data: ph input; R_I_B output; th input; ps input
function R_I_B = calc_R_I_B(ph, th, ps)

R_I_B = [cos(th)*cos(ps)              cos(th)*sin(ps)              -sin(th);
               sin(ph)*sin(th)*cos(ps)-cos(ph)*sin(ps)  sin(ph)*sin(th)*sin(ps)+cos(ph)*cos(ps)  sin(ph)*cos(th);
               cos(ph)*sin(th)*cos(ps)+sin(ph)*sin(ps)  cos(ph)*sin(th)*sin(ps)-sin(ph)*cos(ps)  cos(ph)*cos(th)];
end

== matlab function plant_harness/Subsystem/centreOfPressure1 ==
  data: alpha input; r_L output; phi input; c input; r input; r_R output
function [r_L,r_R] = r_CP(alpha,phi,c,r)

r_L = zeros(3,1);
r_R = zeros(3,1);

% This function generates the distance to the centre of pressure for each
% wing in the wing root frame. This distance is then added to the CG to WR
% distance for each wing to generate the total moment arm. 
%
% The definition of centre of pressure used here is arbitrarily set to be
% the midpoint of the wing. This is an assumption that is expected to be
% improved moving forward, with this script serving as a baseline for
% future work. See the Maple file for more infomation about this
% derivation.

% Left Wing

s = 1;

r_L = [  (1/2)*cos(s*phi)*sin(alpha)*c + (1/2)*sin(s*phi)*s*r ;
        -(1/2)*sin(s*phi)*sin(alpha)*c + (1/2)*cos(s*phi)*s*r ; 
                               -(1/2)*cos(alpha)*c            ;
      ];      

% Right Wing

s = -1;

r_R = [  (1/2)*cos(s*phi)*sin(alpha)*c + (1/2)*sin(s*phi)*s*r ;
        -(1/2)*sin(s*phi)*sin(alpha)*c + (1/2)*cos(s*phi)*s*r ; 
                               -(1/2)*cos(alpha)*c            ;
      ];
      
end
